simulink model "RealTimeProject"  (R2021a)
settings: Solver=FixedStepAuto  StartTime=0.0  StopTime=inf  FixedStep=0.1  RelTol=1e-3  EnableMultiTasking=on
undefined symbols (not defined in the file): PID
libraries: arduinolib x7, simulink x1
settings Model: SILPILModeSetting=veronly  ExtModeTrigDuration=2  Creator=ASUSS  LastModifiedBy=ASUSS
settings OptimizationCC: EnhancedBackFolding=on  PassReuseOutputArgsAs=Individual arguments  ZeroExternalMemoryAtStartup=off  ZeroInternalMemoryAtStartup=off  MaxStackSize=64  OptimizeBlockOrder=speed  DifferentSizesBufferReuse=on  OptimizationCustomize=off  EfficientTunableParamExpr=on
settings DebuggingCC: ParameterTunabilityLossMsg=error
settings HardwareCC: ProdBitPerInt=16  ProdBitPerPointer=16  ProdBitPerSizeT=16  ProdBitPerPtrDiffT=16  ProdLargestAtomicFloat=None  ProdWordSize=8  ProdHWDeviceType=Atmel->AVR  UseEmbeddedCoderFeatures=off
settings SFSimCC: MATLABDynamicMemAlloc=off
settings RTWCC: SystemTargetFile=ert.tlc  HardwareBoard=Arduino Uno  TemplateMakefile=ert_default_tmf  Toolchain=Arduino AVR  BuildConfiguration=Faster Runs
settings CodeAppCC: ForceParamTrailComments=on  IgnoreCustomStorageClasses=off  OperatorAnnotations=on  SimulinkDataObjDesc=on  SFDataObjDesc=on  InsertBlockDesc=on
settings ERTTargetCC: SupportContinuousTime=on  SupportNonInlinedSFcns=on  SupportVariableSizeSignals=on  ExtModeStaticAllocSize=250

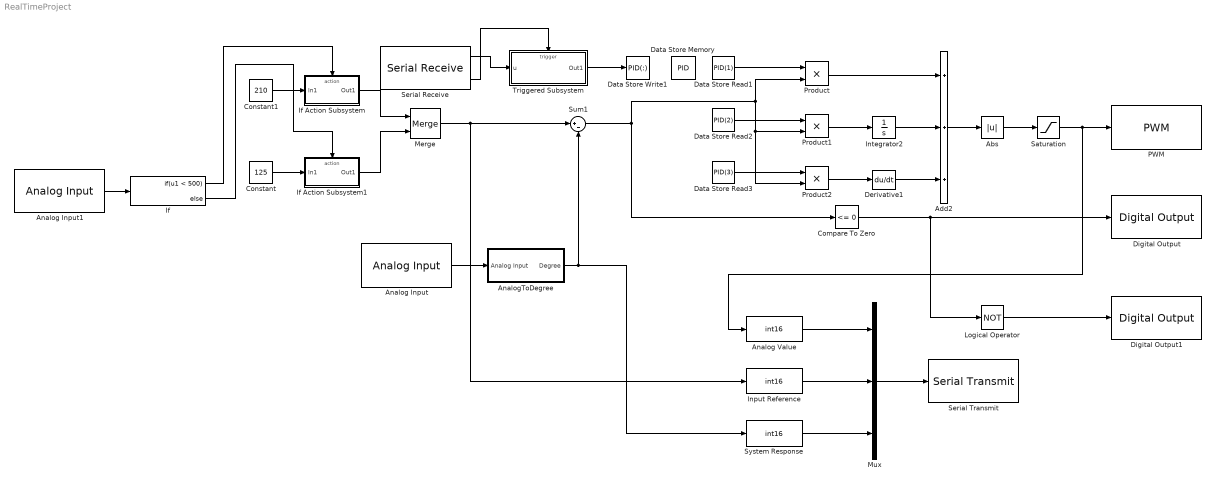
== system RealTimeProject ==
  Abs : Abs
  Add2 : Sum  Inputs=+++
  Analog Input : arduinolib/Analog Input  pinNumber=1  ReadResultsOnly=off  ConversionTriggerSource=Software  ExternalTriggerType=uint32( 0 )  OutputDataType=uint16  EnableConversionCompleteNotify=off  EnableOuputStatus=off  SampleTime=0.1  blockPlatform=arduino
  Analog Input1 : arduinolib/Analog Input  pinNumber=0  ReadResultsOnly=off  ConversionTriggerSource=Software  ExternalTriggerType=uint32( 0 )  OutputDataType=uint16  EnableConversionCompleteNotify=off  EnableOuputStatus=off  SampleTime=0.1  blockPlatform=arduino
  Analog Value : DataTypeConversion  OutDataTypeStr=int16
  AnalogToDegree : Subsystem
  Compare To Zero : simulink/Logic and Bit Operations/Compare To Zero  relop=<=  OutDataTypeStr=boolean
  Constant : Constant  Value=125  SampleTime=0.1
  Constant1 : Constant  Value=210  SampleTime=0.1
  Data Store Memory : DataStoreMemory  DataStoreName=PID  ReadBeforeWriteMsg=warning  WriteAfterWriteMsg=warning  WriteAfterReadMsg=warning  InitialValue=[0 0 0]  ShowAdditionalParam=off
  Data Store Read1 : DataStoreRead  DataStoreName=PID  DataStoreElements=PID(1)  IndexOptions=Index vector (dialog)  Indices=1  OutputSizes=1
  Data Store Read2 : DataStoreRead  DataStoreName=PID  DataStoreElements=PID(2)  IndexOptions=Index vector (dialog)  Indices=1  OutputSizes=1
  Data Store Read3 : DataStoreRead  DataStoreName=PID  DataStoreElements=PID(3)  IndexOptions=Index vector (dialog)  Indices=1  OutputSizes=1
  Data Store Write1 : DataStoreWrite  DataStoreName=PID  DataStoreElements=PID(:)  IndexOptions=Index vector (dialog)  Indices=1  OutputSizes=1
  Derivative1 : Derivative
  Digital Output : arduinolib/Digital Output  pinNumber=9  Direction=output  blockPlatform=arduino
  Digital Output1 : arduinolib/Digital Output  pinNumber=8  Direction=output  blockPlatform=arduino
  If : If  IfExpression=u1 < 500
  If Action Subsystem : Subsystem  TreatAsAtomicUnit=on
  If Action Subsystem1 : Subsystem  TreatAsAtomicUnit=on
  Input Reference : DataTypeConversion  OutDataTypeStr=int16
  Integrator2 : Integrator
  Logical Operator : Logic  Operator=NOT  AllPortsSameDT=off  OutDataTypeStr=boolean
  Merge : Merge
  Mux : Mux  Inputs=3
  PWM : arduinolib/PWM  pinNumber=5  frequencyType=Default  desiredFrequency=490.2  achievableFrequency=490.2
  Product : Product
  Product1 : Product
  Product2 : Product
  Saturation : Saturate  UpperLimit=85  LowerLimit=0
  Serial Receive : arduinolib/Serial Receive  isARMArch=off  portNumber=0  DataType=uint8  Datalength=3  SampleTime=0.1  showOutStatus=on  blockPlatform=arduino
      settings: SourceProductBaseCode=ARDUINO
  Serial Transmit : arduinolib/Serial Transmit  portNumber=0  sendmode=write  sendformat=Decimal  floatprecision=2  blockPlatform=arduino
  Sum1 : Sum  Inputs=|+-
  System Response : DataTypeConversion  OutDataTypeStr=int16
  Triggered Subsystem : Subsystem  TreatAsAtomicUnit=on
  wires:
  Analog Input/1 -> AnalogToDegree/1(Analog Input)
  Analog Input1/1 -> If/1
  Abs/1 -> Saturation/1
  Saturation/1 -> Analog Value/1, PWM/1
  If/1 -> If Action Subsystem/Action
  If/2 -> If Action Subsystem1/Action
  Constant/1 -> If Action Subsystem1/1(In1)
  Constant1/1 -> If Action Subsystem/1(In1)
  If Action Subsystem/1(Out1) -> Merge/1
  If Action Subsystem1/1(Out1) -> Merge/2
  Merge/1 -> Sum1/1, Input Reference/1
  Compare To Zero/1 -> Digital Output/1, Logical Operator/1
  Logical Operator/1 -> Digital Output1/1
  Mux/1 -> Serial Transmit/1
  AnalogToDegree/1(Degree) -> System Response/1, Sum1/2
  Serial Receive/1 -> Triggered Subsystem/1(u)
  Serial Receive/2 -> Triggered Subsystem/Trigger
  Triggered Subsystem/1(Out1) -> Data Store Write1/1
  Sum1/1 -> Compare To Zero/1, Product2/2, Product1/2, Product/2
  Add2/1 -> Abs/1
  Product1/1 -> Integrator2/1
  Derivative1/1 -> Add2/3
  Data Store Read1/1 -> Product/1
  Product/1 -> Add2/1
  Integrator2/1 -> Add2/2
  Product2/1 -> Derivative1/1
  Data Store Read2/1 -> Product1/1
  Data Store Read3/1 -> Product2/1
  Input Reference/1 -> Mux/2
  Analog Value/1 -> Mux/1
  System Response/1 -> Mux/3

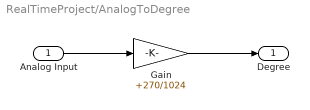
== system RealTimeProject/AnalogToDegree ==
  Analog Input : Inport
  Gain : Gain  Gain=+270/1024
  Degree : Outport
  wires:
  Analog Input/1 -> Gain/1
  Gain/1 -> Degree/1

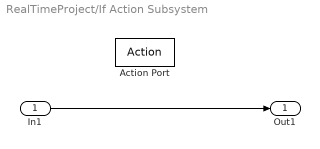
== system RealTimeProject/If Action Subsystem ==
  In1 : Inport
  Action Port : ActionPort  ActionPortLabel=if(u1 < 500)
  Out1 : Outport
  wires:
  In1/1 -> Out1/1

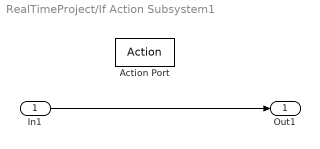
== system RealTimeProject/If Action Subsystem1 ==
  In1 : Inport
  Action Port : ActionPort  ActionPortLabel=else
  Out1 : Outport
  wires:
  In1/1 -> Out1/1

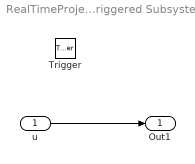
== system RealTimeProject/Triggered Subsystem ==
  u : Inport
  Trigger : TriggerPort  VariantControl=(inherit)
  Out1 : Outport
  wires:
  u/1 -> Out1/1
